simulink model "banking_ndtm"  (R2018b)
settings: configuration reference "Physics" (kept outside this file)
undefined symbols (not defined in the file): VEH__VehicleData__l_WheelbaseF_m, VEH__VehicleData__l_WheelbaseTotal_m, VEH__VehicleData__w_TrackF_m, VEH__VehicleData__w_TrackR_m
settings Model: DataDictionary=vehicleparameters_vehdynsim.sldd  Creator=staer  LastModifiedBy=staer

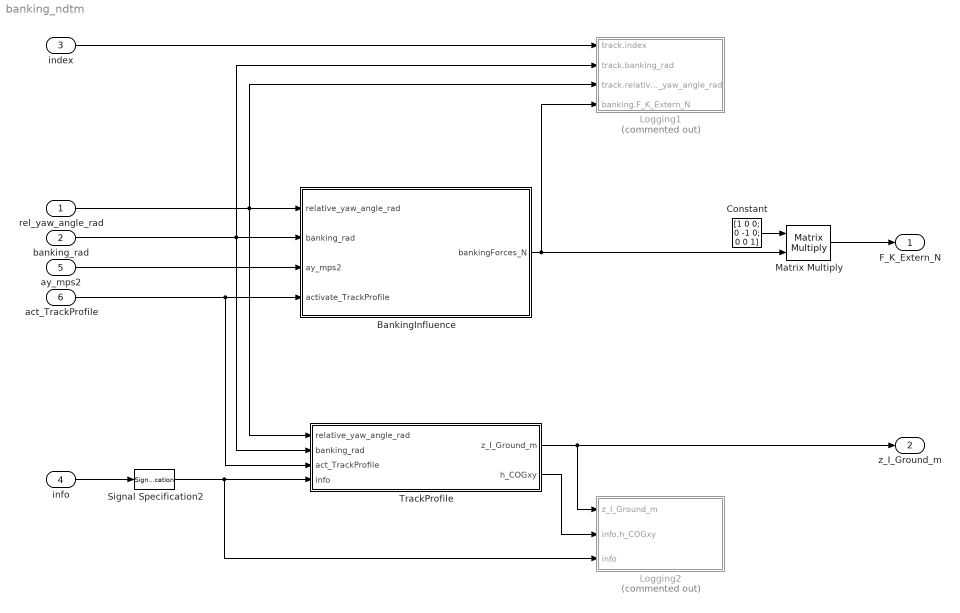
== system banking_ndtm ==
  rel_yaw_angle_rad : Inport
  banking_rad : Inport  Port=2
  index : Inport  Port=3
  info : Inport  Port=4
  ay_mps2 : Inport  Port=5
  act_TrackProfile : Inport  Port=6
  BankingInfluence : MATLAB Function  TreatAsAtomicUnit=on
  Constant : Constant  Value=[1 0 0; 0 -1 0; 0 0 1]
  Logging1 : Subsystem  Commented=on
  Logging2 : Subsystem  Commented=on
  Matrix Multiply : Product  Multiplication=Matrix(*)
  Signal Specification2 : SignalSpecification  Dimensions=[1,4]
  TrackProfile : MATLAB Function  TreatAsAtomicUnit=on
  F_K_Extern_N : Outport
  z_I_Ground_m : Outport  Port=2
  wires:
  info/1 -> Signal Specification2/1
  TrackProfile/1(z_I_Ground_m) -> z_I_Ground_m/1, Logging2/1(z_I_Ground_m)
  BankingInfluence/1(bankingForces_N) -> Matrix Multiply/2, Logging1/4(banking.F_K_Extern_N)
  index/1 -> Logging1/1(track.index)
  ay_mps2/1 -> BankingInfluence/3(ay_mps2)
  TrackProfile/2(h_COGxy) -> Logging2/2(info.h_COGxy)
  banking_rad/1 -> Logging1/2(track.banking_rad), BankingInfluence/2(banking_rad), TrackProfile/2(banking_rad)
  rel_yaw_angle_rad/1 -> Logging1/3(track.relative_yaw_angle_rad), BankingInfluence/1(relative_yaw_angle_rad), TrackProfile/1(relative_yaw_angle_rad)
  act_TrackProfile/1 -> BankingInfluence/4(activate_TrackProfile), TrackProfile/3(act_TrackProfile)
  Signal Specification2/1 -> TrackProfile/4(info), Logging2/3(info)
  Matrix Multiply/1 -> F_K_Extern_N/1
  Constant/1 -> Matrix Multiply/1

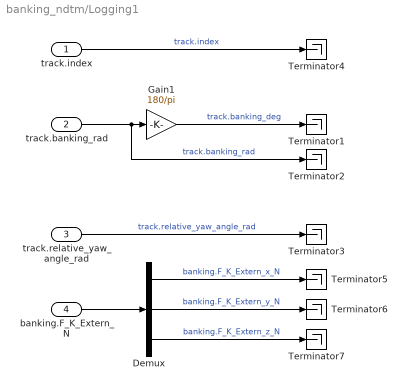
== system banking_ndtm/Logging1 ==
  track.index : Inport
  track.banking_rad : Inport  Port=2
  track.relative_yaw_angle_rad : Inport  Port=3
  banking.F_K_Extern_N : Inport  Port=4
  Demux : Demux  Outputs=3
  Gain1 : Gain  Gain=180/pi
  Terminator{1..7} (7 alike) : Terminator
  wires:
  Gain1/1 -> Terminator1/1  "track.banking_deg"
  track.banking_rad/1 -> Terminator2/1, Gain1/1  "track.banking_rad"
  track.relative_yaw_angle_rad/1 -> Terminator3/1  "track.relative_yaw_angle_rad"
  track.index/1 -> Terminator4/1  "track.index"
  banking.F_K_Extern_N/1 -> Demux/1
  Demux/1 -> Terminator5/1  "banking.F_K_Extern_x_N"
  Demux/2 -> Terminator6/1  "banking.F_K_Extern_y_N"
  Demux/3 -> Terminator7/1  "banking.F_K_Extern_z_N"

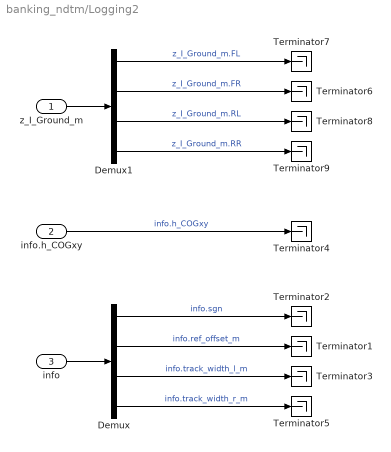
== system banking_ndtm/Logging2 ==
  z_I_Ground_m : Inport
  info.h_COGxy : Inport  Port=2
  info : Inport  Port=3
  Demux : Demux
  Demux1 : Demux
  Terminator{1..9} (9 alike) : Terminator
  wires:
  info/1 -> Demux/1
  Demux/1 -> Terminator2/1  "info.sgn"
  Demux/2 -> Terminator1/1  "info.ref_offset_m"
  Demux/3 -> Terminator3/1  "info.track_width_l_m"
  Demux/4 -> Terminator5/1  "info.track_width_r_m"
  Demux1/4 -> Terminator9/1  "z_I_Ground_m.RR"
  Demux1/3 -> Terminator8/1  "z_I_Ground_m.RL"
  Demux1/2 -> Terminator6/1  "z_I_Ground_m.FR"
  Demux1/1 -> Terminator7/1  "z_I_Ground_m.FL"
  z_I_Ground_m/1 -> Demux1/1
  info.h_COGxy/1 -> Terminator4/1  "info.h_COGxy"

== matlab function banking_ndtm/TrackProfile ==
  data: relative_yaw_angle_rad input; banking_rad input; act_TrackProfile input; z_I_Ground_m output; info input; VEH__VehicleData__l_WheelbaseF_m parameter; h_COGxy output; VEH__VehicleData__l_WheelbaseTotal_m parameter; VEH__VehicleData__w_TrackF_m parameter; VEH__VehicleData__w_TrackR_m parameter
function [z_I_Ground_m, h_COGxy]   = fcn(relative_yaw_angle_rad, banking_rad, act_TrackProfile, info, ...
    VEH__VehicleData__l_WheelbaseF_m, VEH__VehicleData__l_WheelbaseTotal_m, ...
VEH__VehicleData__w_TrackF_m, VEH__VehicleData__w_TrackR_m)

[z_I_Ground_m, h_COGxy] = TrackProfile_ndtm(relative_yaw_angle_rad, banking_rad, act_TrackProfile, info, ...
    VEH__VehicleData__l_WheelbaseF_m, VEH__VehicleData__l_WheelbaseTotal_m, ...
    VEH__VehicleData__w_TrackF_m, VEH__VehicleData__w_TrackR_m);

== matlab function banking_ndtm/BankingInfluence ==
  data: relative_yaw_angle_rad input; banking_rad input; ay_mps2 input; activate_TrackProfile input; bankingForces_N output; VEH__VehicleData__m_Vehicle_kg parameter
function bankingForces_N = fcn(relative_yaw_angle_rad, banking_rad,...
    ay_mps2, activate_TrackProfile, VEH__VehicleData__m_Vehicle_kg)

bankingForces_N = BankingInfluence(relative_yaw_angle_rad, banking_rad,...
    ay_mps2, activate_TrackProfile, VEH__VehicleData__m_Vehicle_kg);
